simulink model "APA_with_PESQ"  (R2024b)
settings: Solver=FixedStepDiscrete  StartTime=0.0  StopTime=inf  RelTol=1e-3  EnableMultiTasking=on
libraries: dspvision x1, dspobslib x1, dspsnks4 x1
settings Model: Creator=The MathWorks, Inc.  LastModifiedBy=HP
settings SolverCC: AlgebraicLoopSolver=TrustRegion  MaxZcPerStep=1
settings DataIOCC: SaveFormat=Array  SaveOutput=off  SaveTime=off  ReturnWorkspaceOutputs=off  SignalLoggingName=sigsOut
settings OptimizationCC: ExpressionDepthLimit=2147483647  InitFltsAndDblsToZero=on  EfficientMapNaN2IntZero=off  LifeSpan=inf  SimCompilerOptimization=on
settings DebuggingCC: UnderspecifiedInitializationDetection=Classic  MergeDetectMultiDrivingBlocksExec=none  CheckExecutionContextPreStartOutputMsg=on  SignalResolutionControl=TryResolveAllWithWarning  MultiTaskDSMMsg=warning  MultiTaskCondExecSysMsg=none  ParameterPrecisionLossMsg=none  FcnCallInpInsideContextMsg=warning  UnconnectedInputMsg=warning  UnconnectedOutputMsg=warning  UnconnectedLineMsg=warning  AllowSymbolicDim=off  StateNameClashWarn=warning  SymbolicDimsDataTypeCodeGenerationDiagnostic=none  SFUnexpectedBacktrackingDiag=warning  SFNoUnconditionalDefaultTransitionDiag=warning  SFExecutionAtInitializationDiag=none  ArithmeticOperatorsInVariantConditions=warning
settings HardwareCC: ProdBitPerPointer=32  ProdBitPerSizeT=32  ProdBitPerPtrDiffT=32  ProdLargestAtomicFloat=None  ProdIntDivRoundTo=Undefined  ProdEndianess=Unspecified  ProdWordSize=32  ProdHWDeviceType=32-bit Generic  TargetUnknown=on
settings ModelReferenceCC: UpdateModelReferenceTargets=IfOutOfDate  EnableRefExpFcnMdlSchedulingChecks=on  PropagateSignalLabelsOutOfModel=off
settings SFSimCC: SimUseLocalCustomCode=off  CustomCodeUndefinedFunction=UseInterfaceOnly
settings RTWCC: RTWUseLocalCustomCode=off  GPUComputeCapability=3.5  DLArmComputeVersion=19.05
settings CodeAppCC: StateflowObjectComments=on
settings GRTTargetCC: TargetFcnLib=ansi_tfl_tmw_new.mat  TargetLangStandard=C89/C90 (ANSI)  CombineOutputUpdateFcns=off  GRTInterface=on
settings ConfigComp: CovMetricSettings=dw  CovSaveCumulativeToWorkspaceVar=on  CovSaveSingleToWorkspaceVar=on  CovExternalEMLEnable=off  CovSFcnEnable=off

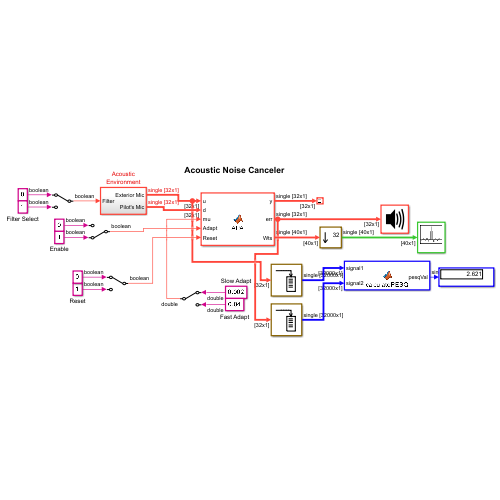
[thumbnail: Simulink's stored preview of the top-level diagram]
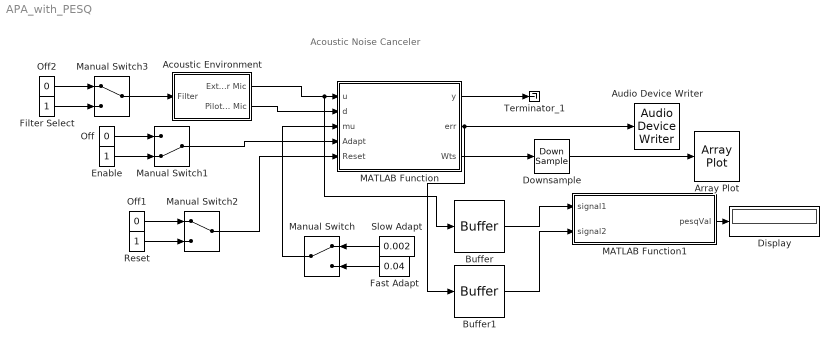
== system APA_with_PESQ ==
  note: Acoustic Noise Canceler
  Acoustic Environment : Subsystem
  Array Plot : ArrayPlot  WindowPosition=[240.000000,133.000000,800.000000,455.000000,]  Visible=on  ScopeFrameLocation=window  XLabel=Samples  YLimits=[-0.075 0.2729]
  Audio Device Writer : dspsnks4/Audio Device Writer  Driver=DirectSound  Device=Default  InheritSampleRate=on  SampleRate=44100  BitDepth=16-bit integer  BufferSize=4096  NumBuffers=10  DefaultOutputChannelMapping=on  OutputChannelMapping=1:2  OutputNumUnderrunSamples=off  DriverIdx=1  DeviceWarnFlag=''
  Buffer : Buffer  N=32000  OutputFrames=off
  Buffer1 : Buffer  N=32000  OutputFrames=off
  Display : Display
  Downsample : DownSample  N=32  RateOptions=Allow multirate processing
  Enable : Constant  OutDataTypeStr=boolean
  Fast Adapt : Constant  Value=0.04  OutDataTypeStr=Inherit: Inherit via back propagation
  Filter Select : Constant  OutDataTypeStr=boolean
  MATLAB Function : MATLAB Function  TreatAsAtomicUnit=on
  MATLAB Function1 : MATLAB Function  TreatAsAtomicUnit=on
  Manual Switch : ManualSwitch
  Manual Switch1 : ManualSwitch  CurrentSetting=0
  Manual Switch2 : ManualSwitch
  Manual Switch3 : ManualSwitch
  Off : Constant  Value=0  OutDataTypeStr=boolean
  Off1 : Constant  Value=0  OutDataTypeStr=boolean
  Off2 : Constant  Value=0  OutDataTypeStr=boolean
  Reset : Constant  OutDataTypeStr=boolean
  Slow Adapt : Constant  Value=0.002  OutDataTypeStr=Inherit: Inherit via back propagation
  Terminator_1 : Terminator
  wires:
  Downsample/1 -> Array Plot/1
  Acoustic Environment/1(Exterior Mic) -> Buffer/1, MATLAB Function/1(u)
  Slow Adapt/1 -> Manual Switch/1
  Fast Adapt/1 -> Manual Switch/2
  Manual Switch/1 -> MATLAB Function/3(mu)
  MATLAB Function/3(Wts) -> Downsample/1
  Acoustic Environment/2(Pilot's Mic) -> MATLAB Function/2(d)
  MATLAB Function/2(err) -> Buffer1/1, Audio Device Writer/1
  MATLAB Function/1(y) -> Terminator_1/1
  Off/1 -> Manual Switch1/1
  Enable/1 -> Manual Switch1/2
  Off1/1 -> Manual Switch2/1
  Reset/1 -> Manual Switch2/2
  Manual Switch1/1 -> MATLAB Function/4(Adapt)
  Manual Switch2/1 -> MATLAB Function/5(Reset)
  Off2/1 -> Manual Switch3/1
  Filter Select/1 -> Manual Switch3/2
  Manual Switch3/1 -> Acoustic Environment/1(Filter)
  MATLAB Function1/1(pesqVal) -> Display/1
  Buffer/1 -> MATLAB Function1/1(signal1)
  Buffer1/1 -> MATLAB Function1/2(signal2)

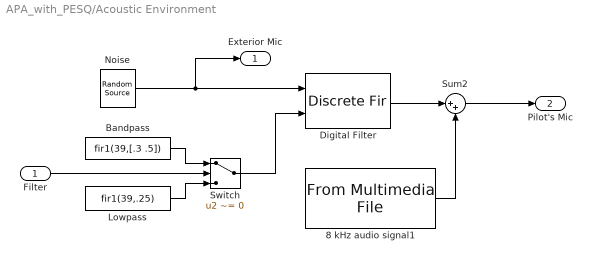
== system APA_with_PESQ/Acoustic Environment ==
  Filter : Inport
  8 kHz audio signal1 : dspvision/From Multimedia File  inputFilename=D:\Advanced Signal Processing\Assignment\output.wav  readRange=[1 Inf]  loop=on  numPlays=inf  outputStreams=Audio only  videoDataType=single  audioDataType=single  inheritSampleTime=on  userDefinedSampleTime=1/30  noAudioOutput=off  isIntensityVideo=off  fourcc=RGB  colorVideoFormat=Separate color signals  outputEOF=off  dataOrg=Column-major  audioFrameSize=32  computeAudioFrameSize=off  outSamplingMode=Sample based
  Bandpass : Constant  Value=fir1(39,[.3 .5])  OutDataTypeStr=Inherit: Inherit via back propagation
  Digital Filter : DiscreteFir  CoefSource=Input port  Coefficients=[1 2]  InputProcessing=Columns as channels (frame based)  AccumDataTypeStr=Inherit: Same as product output  OutDataTypeStr=Inherit: Same as input
      settings: InputPortMap=u0,u1
  Lowpass : Constant  Value=fir1(39,.25)  OutDataTypeStr=Inherit: Inherit via back propagation
  Noise : dspobslib/Random Source  SrcType=Gaussian  NormMethod=Sum of uniform values  CltLength=5  MinVal=-1  MaxVal=1  MeanVal=0  VarVal=1  RepMode=Specify seed  rawSeed=[23341]  IsInherit=off  SampMode=Discrete  SampTime=1/8000  SampFrame=32  DataType=Single  OutComplex=Real  OutputFrames=off
  Sum2 : Sum  Inputs=|++  InputSameDT=on  SaturateOnIntegerOverflow=on  OutDataTypeStr=Inherit: Same as first input
  Switch : Switch  Criteria=u2 ~= 0  InputSameDT=off
  Exterior Mic : Outport  VectorParamsAs1DForOutWhenUnconnected=off
  Pilot's Mic : Outport  Port=2  VectorParamsAs1DForOutWhenUnconnected=off
  wires:
  8 kHz audio signal1/1 -> Sum2/2
  Sum2/1 -> Pilot's Mic/1
  Filter/1 -> Switch/2
  Digital Filter/1 -> Sum2/1
  Noise/1 -> Digital Filter/1, Exterior Mic/1
  Switch/1 -> Digital Filter/2
  Bandpass/1 -> Switch/1
  Lowpass/1 -> Switch/3

== matlab function APA_with_PESQ/MATLAB Function1 ==
  data: signal1 input; pesqVal output; signal2 input
function pesqVal = calculatePESQ(signal1, signal2)
% calculatePESQ calculates an approximate PESQ score between two signals.
% Inputs:
%   signal1 - Reference signal (32x1)
%   signal2 - Degraded signal (32x1)
% Output:
%   pesqVal - Approximated PESQ value (score between 1 and 4.5)
%
% Note: This is a simplified approximation for demonstration purposes.
% The real PESQ algorithm is based on ITU-T P.862 and involves a more
% sophisticated perceptual model.

% Ensure column vectors
signal1 = signal1(:);
signal2 = signal2(:);

% Normalize the signals to avoid scaling issues
signal1 = signal1 / max(abs(signal1) + eps);
signal2 = signal2 / max(abs(signal2) + eps);

% Apply a simple pre-emphasis filter (to mimic some auditory pre-processing)
preemph = [1 -0.95];
sig1_pre = filter(preemph, 1, signal1);
sig2_pre = filter(preemph, 1, signal2);

% Compute FFT for both pre-emphasized signals
N = length(signal1);
S1 = fft(sig1_pre, N);
S2 = fft(sig2_pre, N);

% Use only the first half of the spectrum (real signals)
halfN = floor(N/2);
mag1 = abs(S1(1:halfN));
mag2 = abs(S2(1:halfN));

% Compute the log-spectral distance
logSpecDiff = log10(mag1 + eps) - log10(mag2 + eps);
lsd = sqrt(mean(logSpecDiff.^2));

% Map the log-spectral distance to an approximate PESQ score.
% Here we assume a linear mapping:
% A lower LSD (i.e. smaller error) gives a higher PESQ score.
% Typical PESQ scores range between 1 (poor) and 4.5 (excellent).
pesqVal = 4.5 - (lsd * 2);  % Scale factor chosen for demonstration
pesqVal = max(1, min(4.5, pesqVal)); % Clamp value to [1, 4.5]

end

== matlab function APA_with_PESQ/MATLAB Function ==
  data: u input; y output; err output; Wts output; d input; mu input; Adapt input; Reset input
function [y, err, Wts] = APA(u, d, mu, Adapt, Reset)
% APA - Affine Projection Algorithm implementation for a Simulink MATLAB Function block.
%
% This function implements an adaptive FIR filter with 40 taps.
% The block inputs are:
%   u     - input vector (32x1)
%   d     - desired signal (32x1)
%   mu    - step size (scalar)
%   Adapt - adaptation flag (nonzero enables weight update)
%   Reset - reset flag (nonzero reinitializes the persistent states)
%
% The outputs are:
%   y    - filter output vector (32x1)
%   err  - error vector (desired minus output) (32x1)
%   Wts  - current filter coefficient vector (40x1)
%
% The APA update uses a sliding window of the last P input snapshots and corresponding errors.
% The weight update equation is:
%
%      w(k+1) = w(k) + mu * X_ap * inv(X_ap'*X_ap + delta*I) * e_ap
%
% where:
%   X_ap is the data matrix collecting the most recent P delay-line vectors (size 40xP)
%   e_ap is the corresponding error vector (Px1)

% Initialize persistent variables using the same data type as the input u.
persistent w uBuffer
if isempty(w) || Reset
    w = zeros(40, 1, 'like', u);
end
if isempty(uBuffer) || Reset
    uBuffer = zeros(40, 1, 'like', u);
end

% Number of samples per block (expected to be 32)
N = length(u);  
y   = zeros(N, 1, 'like', u);
err = zeros(N, 1, 'like', u);

% --- APA Parameters ---
P = 8;            % Projection order (number of delay-line snapshots to reuse)
delta = 1e-6;     % Regularization constant (to avoid ill-conditioning)

% Initialize matrices to store delay-line snapshots and corresponding errors.
X_ap = zeros(40, P, 'like', u);
e_ap = zeros(P, 1, 'like', u);

% Process each sample in the input block.
for n = 1:N
    % Update the delay-line: shift the current buffer and insert the new sample at the top.
    uBuffer = [u(n); uBuffer(1:end-1)];
    
    % Compute the filter output as the inner product of weights and the current delay-line.
    y(n) = w' * uBuffer;
    
    % Calculate the error signal (desired minus filter output).
    err(n) = d(n) - y(n);
    
    % Store the current delay-line snapshot and error for APA update.
    if n <= P
        X_ap(:, n) = uBuffer;
        e_ap(n)   = err(n);
    else
        % Use a sliding window: discard the oldest column and add the new one.
        X_ap = [X_ap(:, 2:end), uBuffer];
        e_ap = [e_ap(2:end); err(n)];
    end
end

% If adaptation is enabled and we have at least P samples, update the filter coefficients.
if Adapt && (N >= P)
    % Compute the APA weight update.
    % The term (X_ap'*X_ap + delta*I) is a P x P matrix that is inverted.
    w = w + mu * X_ap * ((X_ap' * X_ap + delta * eye(P, 'like', u)) \ e_ap);
end

% Output the current weight vector.
Wts = w;
end
